simulink model "slowtimemachine"  (R2024a)
settings: Solver=VariableStepAuto  StartTime=0.0  StopTime=100  RelTol=1e-3
model workspace (MAT data in the model file):
  C_load = 0.0001
  Diode_forward_voltage = 1.7
  L_load = 0.01
  R_load = 50
  Threshold_voltage = 5.9
  drain_source_on_resistance = 0.8
  off_state_conductance = 1e-06
  samp_time = 0.00125
  voltage = 50
libraries: ee_lib x10, nesl_utility x9, fl_lib x1, spsTriangleGeneratorLib x1
settings Model: Creator=Konstantin  LastModifiedBy=Konstantin

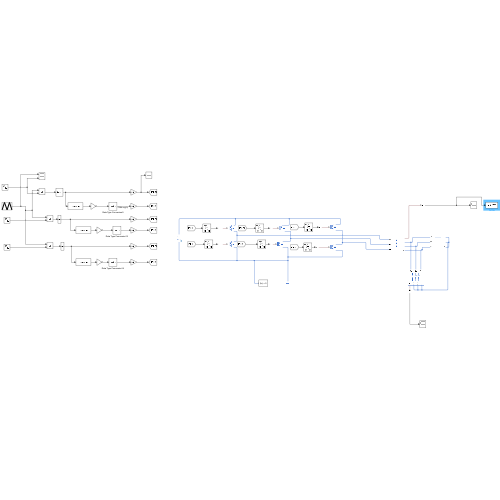
[thumbnail: Simulink's stored preview of the top-level diagram]
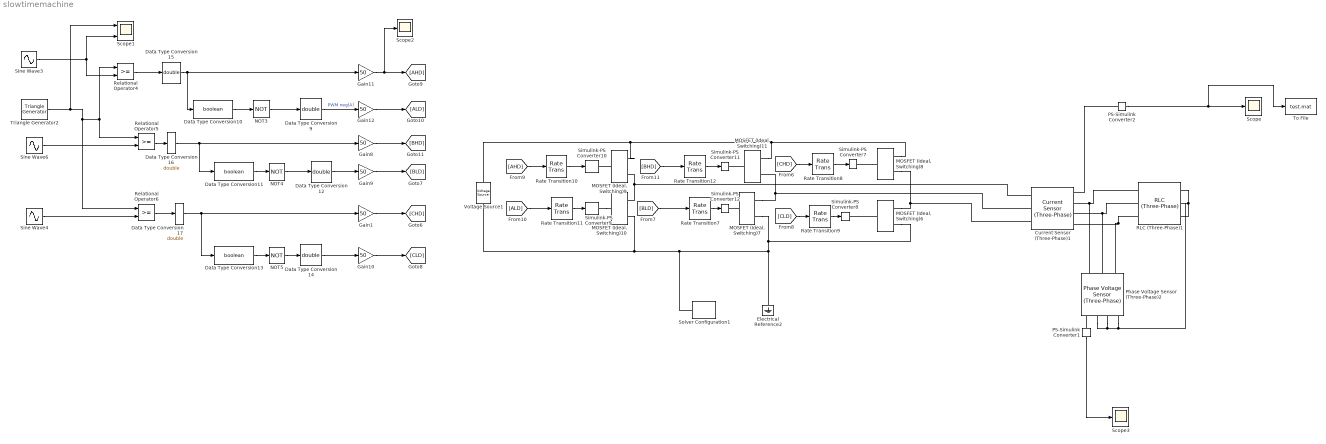
== system slowtimemachine ==
  Current Sensor (Three-Phase)1 : ee_lib/Sensors & Transducers/Current Sensor (Three-Phase)
      settings: InternalSimscapePortConfiguration="{\"Bottom\":[],\"Left\":[{\"id\":\"a1\",\"label\":\"a1\",\"type\":\"foundation.electrical.electrical\"},{\"id\":\"b1\",\"label\":\"b1\",\"type\":\"foundation.electrical.electrical\"},{\"id\":\"c1\",\"label\":\"c1\",\"type\":\"foundation.electrical.electrical\"}],\"Right\":[{\"id\":\"I_output\",\"label\":\"I\",\"type\":\"output\"},{\"id\":\"a2\",\"label\":\"a2\",\"type\":\"foundation.electrical.electrical\"},{\"id\":\"b2\",\"label\":\"b2\",\"type\":\"foundation.electrical.electrical\"},{\"id\":\"c2\",\"label\":\"c2\",\"type\":\"foundation.electrical.electrical\"}],\"Top\":[]}"
  Data Type Conversion10 : DataTypeConversion  OutDataTypeStr=boolean  SaturateOnIntegerOverflow=off  RndMeth=Floor
  Data Type Conversion11 : DataTypeConversion  OutDataTypeStr=boolean  SaturateOnIntegerOverflow=off  RndMeth=Floor
  Data Type Conversion12 : DataTypeConversion  OutDataTypeStr=double  RndMeth=Nearest  SaturateOnIntegerOverflow=off
  Data Type Conversion13 : DataTypeConversion  OutDataTypeStr=boolean  SaturateOnIntegerOverflow=off  RndMeth=Floor
  Data Type Conversion14 : DataTypeConversion  OutDataTypeStr=double  RndMeth=Nearest  SaturateOnIntegerOverflow=off
  Data Type Conversion15 : DataTypeConversion  OutDataTypeStr=double  SaturateOnIntegerOverflow=off  RndMeth=Floor
  Data Type Conversion16 : DataTypeConversion  OutDataTypeStr=double  SaturateOnIntegerOverflow=off  RndMeth=Floor
  Data Type Conversion17 : DataTypeConversion  OutDataTypeStr=double  SaturateOnIntegerOverflow=off  RndMeth=Floor
  Data Type Conversion9 : DataTypeConversion  OutDataTypeStr=double  RndMeth=Nearest  SaturateOnIntegerOverflow=off
  Electrical Reference2 : fl_lib/Electrical/Electrical Elements/Electrical Reference
  Gain{1,8..12} (6 alike) : Gain  Gain=50
  MOSFET (Ideal, Switching){6..11} (6 alike) : ee_lib/Semiconductors & Converters/MOSFET (Ideal, Switching)  port_option=ee.enum.controlport.ps  Rds=0.8 mOhm  Goff=1e-6 1/Ohm  Vth=5.9 V  diode_param=ee.enum.semiconductors.protectionDiode.nodynamics  diode_Vf=1.7 V  diode_Ron=0.001 Ohm  diode_Goff=1e-5 1/Ohm  diode_C=50e-9 F  diode_iRM=-235 A  diode_iF=300 A  diode_idot=-50 A/us  diode_trr_param=ee.enum.converters.diodeReverseParam.trr_factor  diode_trr_factor=3  diode_trr=15 us  diode_Qrr=1500 s*uA  ids_specify=off  ids_priority=None  ids=0 A  ids_nominal_specify=off  ids_nominal_value=1  ids_nominal_unit=A  vds_specify=off  vds_priority=None  vds=0 V  vds_nominal_specify=off  vds_nominal_value=1  vds_nominal_unit=V  vgs_specify=off  vgs_priority=None  vgs=0 V  vgs_nominal_specify=off  vgs_nominal_value=1  vgs_nominal_unit=V  thermal_loss_option=ee.enum.converters.thermalLossOption.constantvalues  Von_data=[0, 1.8, 3.2, 6, 10, 16; 0, 2, 5.5, 9.5, 15, 25] V  Tj=[298.15, 448.15] K  Iout_data=[0, 20, 40, 60, 80, 100] A  Eon_data=[0, 55.04, 124.57, 235.53, 362.12; 0, 71.25, 161.25, 304.88, 468.75] * 1e-6 J  Eoff_data=[0, 18, 30, 56.1, 76.5; 0, 22.5, 37.5, 70.13, 95.63] * 1e-6 J  Eon_data_3D=[zeros(2, 5, 3)] J  Eoff_data_3D=[zeros(2, 5, 3)] J  Tj_loss=[298.15, 448.15] K  Iout_data_loss=[0, 10, 20, 30, 40] A  tabulateWithVds=false  Vds_loss=[0, 150, 300] V  Eon_scalar=22.86e-3 J  Eoff_scalar=17.14e-3 J  Voff=300 V  Iout_scalar=600 A  useCurrentFromPreviousCycle=false  useVoltageFromPreviousCycle=false  diodeModelType=ee.enum.converters.diodeModelType.pwl  diodeTableType=ee.enum.diode.tableType.IfMat  diode_ReverseIVType=ee.enum.diode.diodeReverseIV.constant  diode_IfMat=[.07, .12, .19, 1.75, 4.24, 7.32, 11.2; .16, .3, .72, 2.14, 4.02, 6.35, 9.12] A  diode_VfMat=[.9, 1.15, 1.25, 1.5, 1.75, 2.17, 2.6, 2.85; .58, .68, .75, 1.1, 1.38, 1.77, 2.27, 2.7] V  diode_TjVec=[25, 125] degC  diode_VfVec=[.5, .7, .9, 1.3, 1.7, 2.1, 2.5] V  diode_IfVec=[.1, .2, .5, 1, 2, 4, 7, 10] A  diode_IrMat=[1e-06, 2e-06, 5e-06, 1e-05, 2.5e-05, 5e-05, .0001; 2e-06, 5e-06, 1e-05, 4e-05, 8e-05, .0002, .0005] A  diode_VrMat=[10, 100, 200, 250, 300, 325, 350; 10, 70, 160, 220, 270, 300, 320] V  diode_VrVec=[10, 20, 40, 50, 70, 80, 100] V  diode_IrVec=[1e-06, 2e-06, 5e-06, 1e-05, 2e-05, 5e-05, .0001] A  diode_Vr=-600 V  diode_Ls=150 nH  diode_Erec=0.03 J  diode_rec_loss_model=ee.enum.diode.reverseRecoveryModel.fixed  diode_ErecVal=0 J  diode_scaleWithIandV=true  diode_ErecMat=zeros(2, 3) J  diode_TjrecVec=[298.15, 398.15] K  diode_IfrecVec=[.1, 1, 10] A  diode_IrecVal=10 A  diode_VrecVal=10 V  diode_tFilter=1 / 1000 / 100 s  thermal_network_parameterization=ee.enum.thermalNetworkTopology.external  Rth=[.03, .2] K/W  Rth_Cauer=[.03, .1, .2] K/W  Rth_Foster=[.03, .2] K/W  thermal_mass_parameterization=ee.enum.thermalNetwork.timeconstant  thermal_mass=[3, 25] J/K  thermal_mass_Cauer=[3, 10, 25] J/K  thermal_mass_Foster=[33, 50] J/K  thermal_time_constant=[.1, 5] s  thermal_time_constant_Cauer=[.1, 1, 5] s  thermal_time_constant_Foster=[1, 10] s  thermal_mass_initial_temperatures=[25, 25] degC  thermal_mass_initial_temperatures_Cauer=[25, 25, 25] degC  junction_thermal_mass=0.1 J/K  Tvec_initial_Foster=[25, 25, 25, 25] degC  no_thermal_network=0  junction_temperature_specify=off  junction_temperature_priority=None  junction_temperature=25 degC  junction_temperature_nominal_specify=off  junction_temperature_nominal_value=1  junction_temperature_nominal_unit=degC  Qj_specify=off  Qj_priority=None  Qj=0 W  Qj_nominal_specify=off  Qj_nominal_value=1  Qj_nominal_unit=W  accumulatedSwitchingLosses_specify=off  accumulatedSwitchingLosses_priority=None  accumulatedSwitchingLosses=0 J
  NOT3 : Logic  Operator=NOT  IconShape=distinctive  AllPortsSameDT=off  OutDataTypeStr=boolean
  NOT4 : Logic  Operator=NOT  IconShape=distinctive  AllPortsSameDT=off  OutDataTypeStr=boolean
  NOT5 : Logic  Operator=NOT  IconShape=distinctive  AllPortsSameDT=off  OutDataTypeStr=boolean
  PS-Simulink Converter1 : nesl_utility/PS-Simulink Converter  PhysicalDomain=network_engine_domain  SubClassName=ps_output  LeftPortType=input  RightPortType=output  PseudoPeriodic=off  Frequencies=[]  VectorFormat=inherit  Unit=inherit  AffineConversion=off
  PS-Simulink Converter2 : nesl_utility/PS-Simulink Converter  PhysicalDomain=network_engine_domain  SubClassName=ps_output  LeftPortType=input  RightPortType=output  PseudoPeriodic=off  Frequencies=[]  VectorFormat=inherit  Unit=inherit  AffineConversion=off
  Phase Voltage Sensor (Three-Phase)2 : ee_lib/Sensors & Transducers/Phase Voltage Sensor (Three-Phase)
      settings: InternalSimscapePortConfiguration="{\"Bottom\":[],\"Left\":[{\"id\":\"a1\",\"label\":\"a1\",\"type\":\"foundation.electrical.electrical\"},{\"id\":\"b1\",\"label\":\"b1\",\"type\":\"foundation.electrical.electrical\"},{\"id\":\"c1\",\"label\":\"c1\",\"type\":\"foundation.electrical.electrical\"}],\"Right\":[{\"id\":\"V_output\",\"label\":\"V\",\"type\":\"output\"},{\"id\":\"a2\",\"label\":\"a2\",\"type\":\"foundation.electrical.electrical\"},{\"id\":\"b2\",\"label\":\"b2\",\"type\":\"foundation.electrical.electrical\"},{\"id\":\"c2\",\"label\":\"c2\",\"type\":\"foundation.electrical.electrical\"}],\"Top\":[]}"
  RLC (Three-Phase)1 : ee_lib/Passive/RLC Assemblies/RLC (Three-Phase)  component_structure=ee.enum.rlc.structure.SeriesRLC  R=R_load Ohm  L=L_load*1000 H  C=C_load*1000 F  R_parasitic=0 Ohm  G_parasitic=0 1/Ohm  IL_specify=off  IL_priority=High  IL=[0, 0, 0] A  IL_nominal_specify=off  IL_nominal_value=1  IL_nominal_unit=A  VC_specify=off  VC_priority=High  VC=[0, 0, 0] V  VC_nominal_specify=off  VC_nominal_value=1  VC_nominal_unit=V
      settings: InternalSimscapePortConfiguration="{\"Bottom\":[],\"Left\":[{\"id\":\"a1\",\"label\":\"a1\",\"type\":\"foundation.electrical.electrical\"},{\"id\":\"b1\",\"label\":\"b1\",\"type\":\"foundation.electrical.electrical\"},{\"id\":\"c1\",\"label\":\"c1\",\"type\":\"foundation.electrical.electrical\"}],\"Right\":[{\"id\":\"a2\",\"label\":\"a2\",\"type\":\"foundation.electrical.electrical\"},{\"id\":\"b2\",\"label\":\"b2\",\"type\":\"foundation.electrical.electrical\"},{\"id\":\"c2\",\"label\":\"c2\",\"type\":\"foundation.electrical.electrical\"}],\"Top\":[]}"
  Rate Transition{7..12} (6 alike) : RateTransition
  Relational Operator4 : RelationalOperator  OutDataTypeStr=boolean  RndMeth=Simplest  InputSameDT=off
  Relational Operator5 : RelationalOperator  OutDataTypeStr=boolean  RndMeth=Simplest  InputSameDT=off
  Relational Operator6 : RelationalOperator  OutDataTypeStr=boolean  RndMeth=Simplest  InputSameDT=off
  Scope : Scope
  Scope1 : Scope  NumInputPorts=2
  Scope2 : Scope
  Scope3 : Scope
  Simulink-PS Converter{7..12} (6 alike) : nesl_utility/Simulink-PS Converter  PhysicalDomain=network_engine_domain  SubClassName=ps_input  LeftPortType=input  RightPortType=output  PseudoPeriodic=off  Frequencies=[]  NoiseDistribution=none  NoiseParameters=[]  Unit=1  AffineConversion=off  FilteringAndDerivatives=provide  SimscapeFilterOrder=1  InputFilterTimeConstant=0.001  UdotUserProvided=0
  Sine Wave3 : Sin  Frequency=50*2*pi/2/1000  SampleTime=samp_time
  Sine Wave4 : Sin  Frequency=50*2*pi/2/1000  Phase=4/3*pi  SampleTime=samp_time
  Sine Wave6 : Sin  Frequency=50*2*pi/2/1000  Phase=2/3*pi  SampleTime=samp_time
  Solver Configuration1 : nesl_utility/Solver Configuration  PhysicalDomain=network_engine_domain  SubClassName=solver  LeftPortType=input  RightPortType=generic  Tones=[]  Harmonics=[]  SimulateNoise=off  Profile=off  UseLocalSampling=off  EnableSwitchedLinearOptims=on  FrequencyDomain=off  UseCCode=off  RelTol=0.001  AbsTol=0.001  MinStep=1e-09  ToWorkspace=off  RevertToSquareIcSolve=off  NumHomotopyIterations=100  PhasorMode=off  PhasorModeNumHarmonics=1  ConsistencySolver=NEWTON_XTOL_AFTER_FTOL  IndexReductionMethod=DerivativeReplacement  DoDC=off  ResidualTolerance=1e-09  ConsistencyTolSource=GLOBAL  ConsistencyAbsTol=0.001  ConsistencyRelTol=0.001  ConsistencyTolFactor=0.001  UseLocalSolver=on  LocalSolverChoice=NE_BACKWARD_EULER_ADVANCER  ResolveIndetEquations=on  FunctionEvalNumThread=1  LocalSolverSampleTime=samp_time  DoFixedCost=on  MaxNonlinIter=3  MaxModeIter=2  ComputeImpulses=off  ImpulseIterations=2  LinearAlgebra=auto  LinearAlgebraNumThread=0  EquationFormulation=NE_TIME_EF  DelaysMemoryBudget=1024  AutomaticFiltering=on  FilteringTimeConstant=0.001  PartitionStorageMethod=AS_NEEDED  PartitionMemoryBudget=1024  PartitionMethod=ROBUST  MultibodyUseLocalSolver=off  MultibodyLocalSolverChoice=ODE1  MultibodyLocalSolverSampleTime=0.001
  To File : ToFile  Filename=test.mat  MatrixName=test  SaveFormat=Timeseries
  Triangle Generator2 : spsTriangleGeneratorLib/Triangle Generator  Freq=8000/1000  Phase=0  Ts=samp_time
  Voltage Source1 : ee_lib/Sources/Voltage Source  dc_voltage=voltage V  ac_voltage=0 V  ac_shift=0 rad  ac_frequency=0 Hz  noise_mode=ee.enum.sources.noise.Disabled  PSD=0 V^2/Hz  sample_time=1e-3 s  repeatability=ee.enum.sources.repeatability.NotRepeatable  user_seed=0  auto_seed=572149935  i_specify=off  i_priority=None  i=0 A  i_nominal_specify=off  i_nominal_value=1  i_nominal_unit=A  v_specify=off  v_priority=None  v=0 V  v_nominal_specify=off  v_nominal_value=1  v_nominal_unit=V
      settings: SimscapeInstrumentationLogging=on
  wires:
  [BLD] -> Rate Transition7/1
  Gain9/1 -> [BLD]
  Relational Operator4/1 -> Data Type Conversion15/1
  [AHD] -> Rate Transition10/1
  Gain1/1 -> [CHD]
  Data Type Conversion12/1 -> Gain9/1
  Gain12/1 -> [ALD]
  Gain10/1 -> [CLD]
  [ALD] -> Rate Transition11/1
  Rate Transition11/1 -> Simulink-PS Converter9/1
  [CHD] -> Rate Transition8/1
  NOT3/1 -> Data Type Conversion9/1
  Rate Transition9/1 -> Simulink-PS Converter8/1
  Data Type Conversion14/1 -> Gain10/1
  Relational Operator5/1 -> Data Type Conversion16/1
  Rate Transition7/1 -> Simulink-PS Converter12/1
  [BHD] -> Rate Transition12/1
  Relational Operator6/1 -> Data Type Conversion17/1
  Rate Transition10/1 -> Simulink-PS Converter10/1
  Gain8/1 -> [BHD]
  Data Type Conversion15/1 -> Gain11/1, Data Type Conversion10/1
  Gain11/1 -> Scope2/1, [AHD]
  [CLD] -> Rate Transition9/1
  Sine Wave6/1 -> Relational Operator5/2
  NOT5/1 -> Data Type Conversion14/1
  Triangle Generator2/1 -> Scope1/1, Relational Operator5/1, Relational Operator4/1, Relational Operator6/1
  Data Type Conversion13/1 -> NOT5/1
  NOT4/1 -> Data Type Conversion12/1
  PS-Simulink Converter1/1 -> Scope3/1
  Data Type Conversion16/1 -> Gain8/1, Data Type Conversion11/1
  Data Type Conversion17/1 -> Gain1/1, Data Type Conversion13/1
  Rate Transition12/1 -> Simulink-PS Converter11/1
  Sine Wave4/1 -> Relational Operator6/2
  Data Type Conversion11/1 -> NOT4/1
  Data Type Conversion10/1 -> NOT3/1
  Data Type Conversion9/1 -> Gain12/1  "PWM neg(A)"
  Sine Wave3/1 -> Relational Operator4/2, Scope1/2
  Rate Transition8/1 -> Simulink-PS Converter7/1
  PS-Simulink Converter2/1 -> To File/1, Scope/1
  connections:
  RLC (Three-Phase)1/LConn3 -- Phase Voltage Sensor (Three-Phase)2/LConn3 -- Current Sensor (Three-Phase)1/RConn4
  Voltage Source1/RConn1 -- "MOSFET (Ideal, Switching)10"/RConn2 -- Solver Configuration1/RConn1 -- "MOSFET (Ideal, Switching)6"/RConn2 -- "MOSFET (Ideal, Switching)7"/RConn2 -- Electrical Reference2/LConn1
  RLC (Three-Phase)1/LConn1 -- Phase Voltage Sensor (Three-Phase)2/LConn1 -- Current Sensor (Three-Phase)1/RConn2
  RLC (Three-Phase)1/LConn2 -- Phase Voltage Sensor (Three-Phase)2/LConn2 -- Current Sensor (Three-Phase)1/RConn3
  "MOSFET (Ideal, Switching)7"/RConn1 -- Current Sensor (Three-Phase)1/LConn2 -- "MOSFET (Ideal, Switching)11"/RConn2
  "MOSFET (Ideal, Switching)6"/RConn1 -- "MOSFET (Ideal, Switching)8"/RConn2 -- Current Sensor (Three-Phase)1/LConn3
  "MOSFET (Ideal, Switching)9"/RConn1 -- Voltage Source1/LConn1 -- "MOSFET (Ideal, Switching)8"/RConn1 -- "MOSFET (Ideal, Switching)11"/RConn1
  Phase Voltage Sensor (Three-Phase)2/RConn3 -- RLC (Three-Phase)1/RConn2 -- RLC (Three-Phase)1/RConn3 -- RLC (Three-Phase)1/RConn1 -- Phase Voltage Sensor (Three-Phase)2/RConn4 -- Phase Voltage Sensor (Three-Phase)2/RConn2
  "MOSFET (Ideal, Switching)9"/RConn2 -- Current Sensor (Three-Phase)1/LConn1 -- "MOSFET (Ideal, Switching)10"/RConn1
  PS-Simulink Converter2/LConn1 -- Current Sensor (Three-Phase)1/RConn1
  "MOSFET (Ideal, Switching)6"/LConn1 -- Simulink-PS Converter8/RConn1
  "MOSFET (Ideal, Switching)9"/LConn1 -- Simulink-PS Converter10/RConn1
  "MOSFET (Ideal, Switching)8"/LConn1 -- Simulink-PS Converter7/RConn1
  PS-Simulink Converter1/LConn1 -- Phase Voltage Sensor (Three-Phase)2/RConn1
  "MOSFET (Ideal, Switching)7"/LConn1 -- Simulink-PS Converter12/RConn1
  Simulink-PS Converter9/RConn1 -- "MOSFET (Ideal, Switching)10"/LConn1
  "MOSFET (Ideal, Switching)11"/LConn1 -- Simulink-PS Converter11/RConn1
